simulink model "hierarchical_model"  (R2024a)
settings: Solver=FixedStepAuto  StartTime=0.0  StopTime=10.0  FixedStep=0.1  RelTol=1e-3
settings Model: Creator=amir  LastModifiedBy=amir

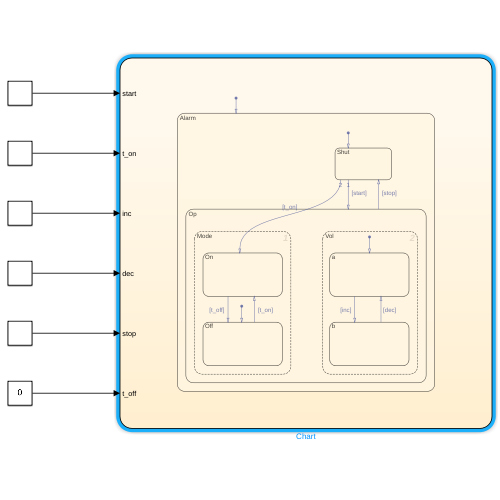
[thumbnail: Simulink's stored preview of the top-level diagram]
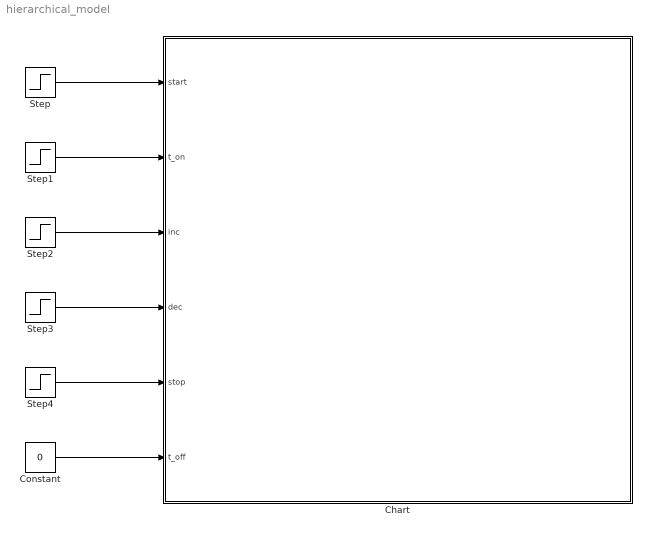
== system hierarchical_model ==
  Chart : Stateflow chart  TreatAsAtomicUnit=on
  Constant : Constant  Value=0
  Step : Step  SampleTime=0
  Step1 : Step  Time=1.1  SampleTime=0
  Step2 : Step  Time=1.2  SampleTime=0
  Step3 : Step  Time=1.3  SampleTime=0
  Step4 : Step  Time=1.4  SampleTime=0
  wires:
  Step/1 -> Chart/1(start)
  Step1/1 -> Chart/2(t_on)
  Step2/1 -> Chart/3(inc)
  Step3/1 -> Chart/4(dec)
  Step4/1 -> Chart/5(stop)
  Constant/1 -> Chart/6(t_off)

== stateflow chart hierarchical_model/Chart ==
  state Alarm
    state Shut
    state Op
      state Mode [parallel]
        settings: executionOrder=1
        state On
        state Off
        On -> Off : [t_off]
        Off -> On : [t_on]
        (default) -> Off
      state Vol [parallel]
        settings: executionOrder=2
        state a
        state b
        (default) -> a
        a -> b : [inc]
        b -> a : [dec]
    (default) -> Shut
    Shut -> On [order 2] : [t_on]
    Shut -> Op [order 1] : [start]
    Op -> Shut : [stop]
  (default) -> Alarm
  data: start input; t_on input; inc input; dec input; stop input; t_off input
